simulink model "sim_fbk"  (R2019b)
settings: Solver=ode4  StartTime=0.0  StopTime=16  FixedStep=0.001  RelTol=1e-3
settings Model: Creator=kawata  LastModifiedBy=kawata
settings DataIOCC: ReturnWorkspaceOutputs=off
settings DebuggingCC: ArithmeticOperatorsInVariantConditions=warning
settings SFSimCC: SimUseLocalCustomCode=off  CustomCodeUndefinedFunction=UseInterfaceOnly
settings RTWCC: RTWUseLocalCustomCode=off

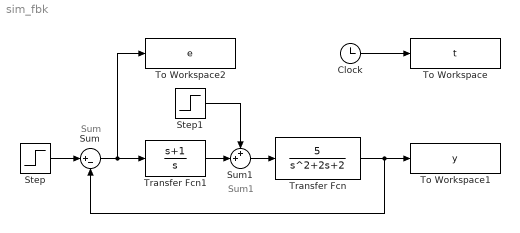
== system sim_fbk ==
  note: Sum1
  note: Sum
  Clock : Clock
  Step : Step  Time=0  SampleTime=0
  Step1 : Step  Time=8  SampleTime=0
  Sum : Sum  Inputs=|+-
  Sum1 : Sum  Inputs=++|
  To Workspace : ToWorkspace  VariableName=t  SampleTime=-1
  To Workspace1 : ToWorkspace  VariableName=y  SampleTime=-1
  To Workspace2 : ToWorkspace  VariableName=e  SampleTime=-1
  Transfer Fcn : TransferFcn  Numerator=[5]  Denominator=[1 2 2]
  Transfer Fcn1 : TransferFcn  Numerator=[1 1]  Denominator=[1 0]
  wires:
  Sum1/1 -> Transfer Fcn/1
  Transfer Fcn/1 -> To Workspace1/1, Sum/2
  Clock/1 -> To Workspace/1
  Step1/1 -> Sum1/1
  Transfer Fcn1/1 -> Sum1/2
  Sum/1 -> To Workspace2/1, Transfer Fcn1/1
  Step/1 -> Sum/1
